simulink model "SIM_NARENDRA_1_METODO_INVERSA_THETA_P_DENTRO_FECHO"  (R2015a)
settings: Solver=ode3  StartTime=0.0  StopTime=40  FixedStep=1e-4  RelTol=1e-3
settings Model: Creator=user  LastModifiedBy=user

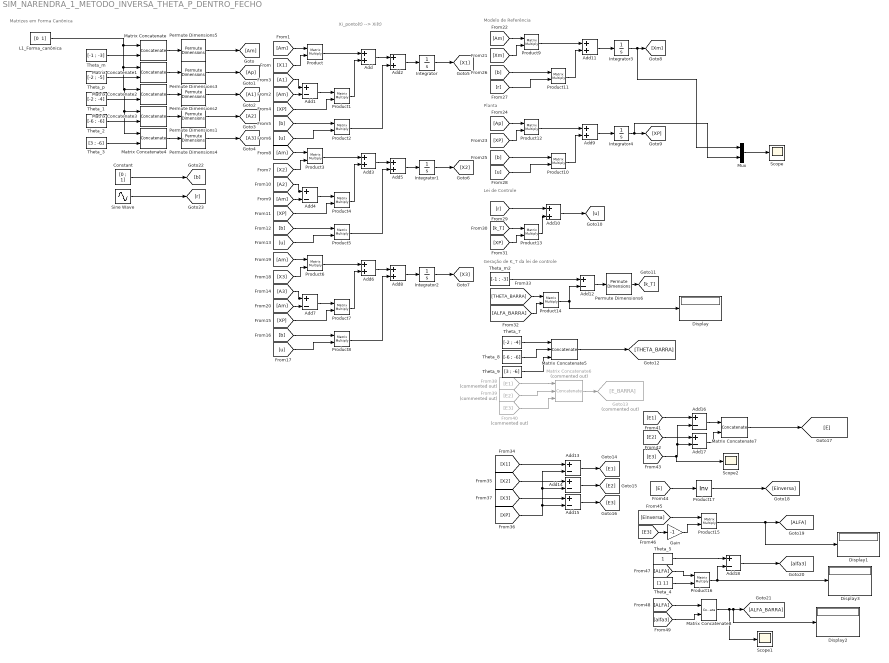
== system SIM_NARENDRA_1_METODO_INVERSA_THETA_P_DENTRO_FECHO ==
  note: Geração de K_T da lei de controle
  note: Lei de Controle
  note: Planta
  note: Modelo de Referência
  note: Matrizes em Forma Canônica
  note: Xi_ponto(t) --> Xi(t)
  Add{,2..3,5..6,8..11} (9 alike) : Sum
  Add{1,4,7,12..18} (10 alike) : Sum  Inputs=+-
  Constant : Constant  Value=[0 ; 1]
  Display{,1..3} (4 alike) : Display
  From38 : From  Commented=on  GotoTag=E1
  From39 : From  Commented=on  GotoTag=E2
  From40 : From  Commented=on  GotoTag=E3
  Gain : Gain  Gain=-1
  Goto13 : Goto  Commented=on  GotoTag=E_BARRA
  Integrator : Integrator  InitialCondition=[2 2]
  Integrator1 : Integrator  InitialCondition=[1 0]
  Integrator2 : Integrator  InitialCondition=[0 0]
  Integrator3 : Integrator
  Integrator4 : Integrator  InitialCondition=[0.01 0.02]
  L1_Forma_canônica : Constant  Value="[0  1]"
  Matrix Concatenate{,1..4,7} (6 alike) : Concatenate  Mode=Multidimensional array  ConcatenateDimension=2
  Matrix Concatenate5 : Concatenate  NumInputs=3  Mode=Multidimensional array  ConcatenateDimension=2
  Matrix Concatenate6 : Concatenate  Commented=on  NumInputs=3  Mode=Multidimensional array  ConcatenateDimension=2
  Matrix Concatenate8 : Concatenate
  Mux : Mux  Inputs=2
  Permute Dimensions{1..6} (6 alike) : PermuteDimensions
  Product{,1..16} (17 alike) : Product  Multiplication=Matrix(*)
  Product17 : Product  Inputs=/  Multiplication=Matrix(*)
  Scope : Scope
      settings: YMin=-0.05  YMax=1
  Scope1 : Scope
      settings: YMin=-2250  YMax=2500
  Scope2 : Scope
      settings: YMin=-0.5  YMax=5.5  SaveName=ScopeData2
  Sine Wave : Sin  Amplitude=0.1  Bias=1  SampleTime=0
  Theta_1 : Constant  Value=[-2 ; -4]
  Theta_2 : Constant  Value=[-6 ; -6]
  Theta_3 : Constant  Value=[3 ; -6]
  Theta_4 : Constant  Value=[1 1]
  Theta_5 : Constant
  Theta_7 : Constant  Value=[-2 ; -4]
  Theta_8 : Constant  Value=[-6 ; -6]
  Theta_9 : Constant  Value=[3 ; -6]
  Theta_m : Constant  Value=[-1 ; -3]
  Theta_m2 : Constant  Value=[-1 ; -3]
  Theta_p : Constant  Value=[-2 ; -5]
  wires:
  Theta_m/1 -> Matrix Concatenate/2
  L1_Forma_canônica/1 -> Matrix Concatenate4/1, Matrix Concatenate3/1, Matrix Concatenate2/1, Matrix Concatenate1/1, Matrix Concatenate/1
  Theta_p/1 -> Matrix Concatenate1/2
  Theta_1/1 -> Matrix Concatenate2/2
  Theta_2/1 -> Matrix Concatenate3/2
  Theta_3/1 -> Matrix Concatenate4/2
  Matrix Concatenate/1 -> Permute Dimensions5/1
  Matrix Concatenate1/1 -> Permute Dimensions3/1
  Matrix Concatenate2/1 -> Permute Dimensions2/1
  Matrix Concatenate3/1 -> Permute Dimensions1/1
  Matrix Concatenate4/1 -> Permute Dimensions4/1
  Permute Dimensions4/1 -> [A3]
  Permute Dimensions1/1 -> [A2]
  Permute Dimensions2/1 -> [A1]
  Permute Dimensions3/1 -> [Ap]
  Permute Dimensions5/1 -> [Am]
  [Am] -> Product/1
  [X1] -> Product/2
  Product/1 -> Add/1
  Product1/1 -> Add/2
  Add1/1 -> Product1/1
  [Am] -> Add1/2
  [A1] -> Add1/1
  [XP] -> Product1/2
  Add/1 -> Add2/1
  Product2/1 -> Add2/2
  [b] -> Product2/1
  [u] -> Product2/2
  Add2/1 -> Integrator/1
  Integrator/1 -> [X1]
  [Am] -> Product3/1
  [X2] -> Product3/2
  Product3/1 -> Add3/1
  Product4/1 -> Add3/2
  Add4/1 -> Product4/1
  [Am] -> Add4/2
  [A2] -> Add4/1
  [XP] -> Product4/2
  Add3/1 -> Add5/1
  Product5/1 -> Add5/2
  [b] -> Product5/1
  [u] -> Product5/2
  Add5/1 -> Integrator1/1
  Integrator1/1 -> [X2]
  [X3] -> Product6/2
  Product6/1 -> Add6/1
  Product7/1 -> Add6/2
  Add7/1 -> Product7/1
  [Am] -> Add7/2
  [A3] -> Add7/1
  [XP] -> Product7/2
  Add6/1 -> Add8/1
  Product8/1 -> Add8/2
  [b] -> Product8/1
  [u] -> Product8/2
  Add8/1 -> Integrator2/1
  Integrator2/1 -> [X3]
  [Am] -> Product6/1
  [Xm] -> Product9/2
  Product9/1 -> Add11/1
  Product11/1 -> Add11/2
  [b] -> Product11/1
  [r] -> Product11/2
  Add11/1 -> Integrator3/1
  [Am] -> Product9/1
  [XP] -> Product12/2
  Product12/1 -> Add9/1
  Product10/1 -> Add9/2
  [b] -> Product10/1
  [u] -> Product10/2
  Add9/1 -> Integrator4/1
  Integrator4/1 -> Mux/2, [XP]
  [Ap] -> Product12/1
  [k_T] -> Product13/1
  [XP] -> Product13/2
  Product13/1 -> Add10/2
  [r] -> Add10/1
  Add10/1 -> [u]
  Permute Dimensions6/1 -> [k_T]
  [THETA_BARRA] -> Product14/1
  [ALFA_BARRA] -> Product14/2
  Theta_m2/1 -> Add12/1
  Product14/1 -> Display/1, Add12/2
  Add12/1 -> Permute Dimensions6/1
  Theta_7/1 -> Matrix Concatenate5/1
  Theta_8/1 -> Matrix Concatenate5/2
  Theta_9/1 -> Matrix Concatenate5/3
  Matrix Concatenate5/1 -> [THETA_BARRA]
  [X1] -> Add13/1
  [XP] -> Add15/2, Add14/2, Add13/2
  [X2] -> Add14/1
  [X3] -> Add15/1
  Add13/1 -> [E1]
  Add14/1 -> [E2]
  Add15/1 -> [E3]
  Matrix Concatenate6/1 -> Goto13/1
  From38/1 -> Matrix Concatenate6/1
  From39/1 -> Matrix Concatenate6/2
  From40/1 -> Matrix Concatenate6/3
  [E3] -> Scope2/1, Add17/2, Add16/2
  [E1] -> Add16/1
  [E2] -> Add17/1
  Add17/1 -> Matrix Concatenate7/2
  Add16/1 -> Matrix Concatenate7/1
  [E] -> Product17/1
  [Einversa] -> Product15/1
  [E3] -> Gain/1
  [ALFA] -> Product16/1
  Theta_4/1 -> Product16/2
  Theta_5/1 -> Add18/1
  Product16/1 -> Display3/1, Add18/2
  [ALFA] -> Matrix Concatenate8/1
  [alfa3] -> Matrix Concatenate8/2
  Matrix Concatenate8/1 -> Scope1/1, Display2/1, [ALFA_BARRA]
  Constant/1 -> [b]
  Sine Wave/1 -> [r]
  Matrix Concatenate7/1 -> [E]
  Product17/1 -> [Einversa]
  Integrator3/1 -> Mux/1, [Xm]
  Mux/1 -> Scope/1
  Product15/1 -> Display1/1, [ALFA]
  Add18/1 -> [alfa3]
  Gain/1 -> Product15/2
